simulink library "transformer_lib"  (Simulink 7.8)
settings: Solver=ode45  StartTime=0.0  StopTime=10.0  RelTol=1e-3
undefined symbols (not defined in the file or in its folder): D1, Delta
libraries: powerlib x15
settings Model: Creator=mi24996  LastModifiedBy=RE25624

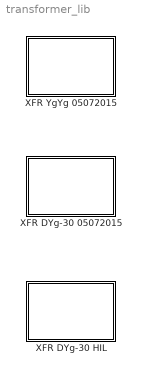
== system transformer_lib ==
  XFR DYg-30 05072015 : Subsystem  mask{Rating=25E3, Vp=12.47E3, Vs=480, Rpu=0.004, Xpu=0.02}
      mask prompts: Rating "Rating [VA]"; Vp "Primary Voltage [VRMSLL]"; Vs "Secondary Voltage [VRMSLL]"; Rpu "Resistance [p.u.]"; Xpu "Reactance [p.u.]"
  XFR DYg-30 HIL : Subsystem  mask(Transformers){Rating=225, Vp=4160, Vs=208, Z=5.18, XR=2.5}
      mask prompts: Rating "Rating [kVA]"; Vp "Primary Voltage [VRMSLL]"; Vs "Secondary Voltage [VRMSLL]"; Z "Impedance, Z [%]"; XR "X/R Ratio"
      mask help:
      | The distribution transformer is implemented using three single-phase transformers connected D/Ygrounded with a negative 30 degrees angular displacement, and operated with fixed turn ratios.
      | The connectivity convention of this block is as follows: ABC indicates the “primary” or high voltage side, and the abc indicates the “secondary” or low voltage side.
  XFR YgYg 05072015 : Subsystem  mask{Rating=25E3, Vp=12.47E3, Vs=480, Rpu=0.004, Xpu=0.02}
      mask prompts: Rating "Rating [VA]"; Vp "Primary Voltage [VRMSLL]"; Vs "Secondary Voltage [VRMSLL]"; Rpu "Resistance [p.u.]"; Xpu "Reactance [p.u.]"

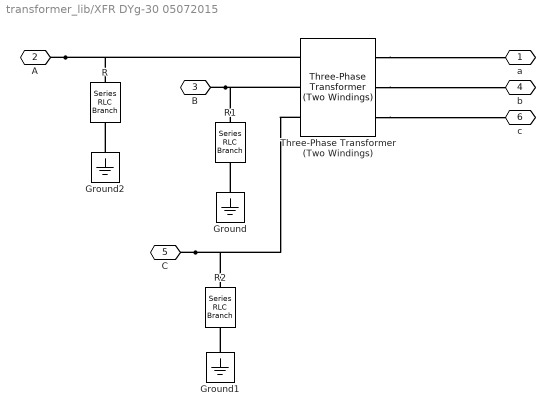
== system transformer_lib/XFR DYg-30 05072015 ==
  Ground : powerlib/Elements/Ground  LConnTagsString=a
  Ground1 : powerlib/Elements/Ground  LConnTagsString=a
  Ground2 : powerlib/Elements/Ground  LConnTagsString=a
  R : powerlib/Elements/Series RLC Branch  LConnTagsString=__new0  RConnTagsString=__new0  BranchType=R  Resistance=10E6  Inductance=0  SetiL0=off  InitialCurrent=0  Capacitance=0  Setx0=off  InitialVoltage=0  Measurements=None
  R1 : powerlib/Elements/Series RLC Branch  LConnTagsString=__new0  RConnTagsString=__new0  BranchType=R  Resistance=10E6  Inductance=0  SetiL0=off  InitialCurrent=0  Capacitance=0  Setx0=off  InitialVoltage=0  Measurements=None
  R2 : powerlib/Elements/Series RLC Branch  LConnTagsString=__new0  RConnTagsString=__new0  BranchType=R  Resistance=10E6  Inductance=0  SetiL0=off  InitialCurrent=0  Capacitance=0  Setx0=off  InitialVoltage=0  Measurements=None
  Three-Phase Transformer (Two Windings) : powerlib/Elements/Three-Phase Transformer (Two Windings)  Winding1Connection=Delta (D1)  UNITS=pu  NominalPower=[ Rating , 60 ]  Winding1=[ Vp , 0 , 0]  Winding2Connection=Yg  Winding2=[ Vs , Rpu, Xpu/(2*pi*60) ]  SetSaturation=off  Rm=500  Lm=500  Saturation=[ 0,0 ; 0.0024,1.2 ; 1.0,1.52 ]  Hysteresis=off  DataFile='hysteresis'  SetInitialFlux=off  InitialFluxes=[ 0.8 , -0.8 , 0.7 ]  Measurements=None  MoreParameters=off  BreakLoop=off  DataType=off  TransfoNumber=1
  a : PMIOPort  Port=1  Side=Right
  A : PMIOPort  Port=2  Side=Left
  B : PMIOPort  Port=3  Side=Left
  b : PMIOPort  Port=4  Side=Right
  C : PMIOPort  Port=5  Side=Left
  c : PMIOPort  Port=6  Side=Right
  connections:
  Ground1/LConn1 -- R2/RConn1
  Ground/LConn1 -- R1/RConn1
  Ground2/LConn1 -- R/RConn1
  Three-Phase Transformer (Two Windings)/RConn2 -- b/RConn1
  C/RConn1 -- R2/LConn1 -- Three-Phase Transformer (Two Windings)/LConn3
  Three-Phase Transformer (Two Windings)/RConn1 -- a/RConn1
  Three-Phase Transformer (Two Windings)/RConn3 -- c/RConn1
  B/RConn1 -- Three-Phase Transformer (Two Windings)/LConn2 -- R1/LConn1
  A/RConn1 -- R/LConn1 -- Three-Phase Transformer (Two Windings)/LConn1

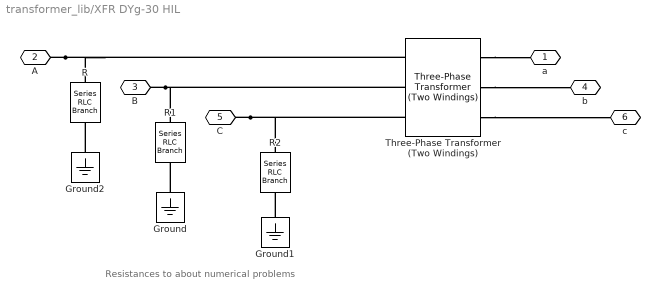
== system transformer_lib/XFR DYg-30 HIL ==
  note: Resistances to about numerical problems
  Ground : powerlib/Elements/Ground  LConnTagsString=a
  Ground1 : powerlib/Elements/Ground  LConnTagsString=a
  Ground2 : powerlib/Elements/Ground  LConnTagsString=a
  R : powerlib/Elements/Series RLC Branch  LConnTagsString=__new0  RConnTagsString=__new0  BranchType=R  Resistance=5E6  Inductance=0  SetiL0=off  InitialCurrent=0  Capacitance=0  Setx0=off  InitialVoltage=0  Measurements=None
  R1 : powerlib/Elements/Series RLC Branch  LConnTagsString=__new0  RConnTagsString=__new0  BranchType=R  Resistance=5E6  Inductance=0  SetiL0=off  InitialCurrent=0  Capacitance=0  Setx0=off  InitialVoltage=0  Measurements=None
  R2 : powerlib/Elements/Series RLC Branch  LConnTagsString=__new0  RConnTagsString=__new0  BranchType=R  Resistance=5E6  Inductance=0  SetiL0=off  InitialCurrent=0  Capacitance=0  Setx0=off  InitialVoltage=0  Measurements=None
  Three-Phase Transformer (Two Windings) : powerlib/Elements/Three-Phase Transformer (Two Windings)  Winding1Connection=Delta (D1)  UNITS=pu  NominalPower=[ Rating*1E3 , 60 ]  Winding1=[ Vp , 0 , 0]  Winding2Connection=Yg  Winding2=[ Vs , Z/(100*XR) , Z/(2*pi*60*100) ]  SetSaturation=off  Rm=500  Lm=500  Saturation=[ 0,0 ; 0.0024,1.2 ; 1.0,1.52 ]  Hysteresis=off  DataFile='hysteresis'  SetInitialFlux=off  InitialFluxes=[ 0.8 , -0.8 , 0.7 ]  Measurements=None  MoreParameters=off  BreakLoop=off  DataType=off  TransfoNumber=1
  a : PMIOPort  Port=1  Side=Right
  A : PMIOPort  Port=2  Side=Left
  B : PMIOPort  Port=3  Side=Left
  b : PMIOPort  Port=4  Side=Right
  C : PMIOPort  Port=5  Side=Left
  c : PMIOPort  Port=6  Side=Right
  connections:
  Ground1/LConn1 -- R2/RConn1
  Ground/LConn1 -- R1/RConn1
  Ground2/LConn1 -- R/RConn1
  Three-Phase Transformer (Two Windings)/RConn2 -- b/RConn1
  C/RConn1 -- R2/LConn1 -- Three-Phase Transformer (Two Windings)/LConn3
  Three-Phase Transformer (Two Windings)/RConn1 -- a/RConn1
  Three-Phase Transformer (Two Windings)/RConn3 -- c/RConn1
  B/RConn1 -- Three-Phase Transformer (Two Windings)/LConn2 -- R1/LConn1
  A/RConn1 -- R/LConn1 -- Three-Phase Transformer (Two Windings)/LConn1

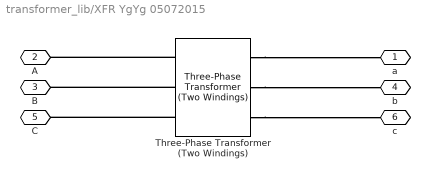
== system transformer_lib/XFR YgYg 05072015 ==
  Three-Phase Transformer (Two Windings) : powerlib/Elements/Three-Phase Transformer (Two Windings)  Winding1Connection=Yg  UNITS=pu  NominalPower=[ Rating , 60 ]  Winding1=[ Vp , 0 , 0]  Winding2Connection=Yg  Winding2=[ Vs , Rpu , Xpu/(2*pi*60) ]  SetSaturation=off  Rm=500  Lm=500  Saturation=[ 0,0 ; 0.0024,1.2 ; 1.0,1.52 ]  Hysteresis=off  DataFile='hysteresis'  SetInitialFlux=off  InitialFluxes=[ 0.8 , -0.8 , 0.7 ]  Measurements=None  MoreParameters=off  BreakLoop=off  DataType=off  TransfoNumber=1
  a : PMIOPort  Port=1  Side=Right
  A : PMIOPort  Port=2  Side=Left
  B : PMIOPort  Port=3  Side=Left
  b : PMIOPort  Port=4  Side=Right
  C : PMIOPort  Port=5  Side=Left
  c : PMIOPort  Port=6  Side=Right
  connections:
  Three-Phase Transformer (Two Windings)/RConn2 -- b/RConn1
  Three-Phase Transformer (Two Windings)/LConn3 -- C/RConn1
  Three-Phase Transformer (Two Windings)/RConn1 -- a/RConn1
  Three-Phase Transformer (Two Windings)/RConn3 -- c/RConn1
  Three-Phase Transformer (Two Windings)/LConn2 -- B/RConn1
  Three-Phase Transformer (Two Windings)/LConn1 -- A/RConn1
